simulink model "modello_completo_simulink2018b"  (R2018b)
settings: Solver=VariableStepAuto  StartTime=0.0  StopTime=10  RelTol=1e-3
undefined symbols (not defined in the file): a1, a2, AHRS_bias, AHRS_sample_time, AHRS_var, alpha1, alpha2, c, current, D, dead_zone_limit, DVL_sample_t, DVL_var1, DVL_var2, DVL_var3, gps_sample_t, IMU_sample_time, initial, M, M_inv, n_max, omega, ps_sample_t, ps_sample_t2, ps_var, ps_var2, pylonCenter, pylonRadius, rho, s_data, TAM
libraries: simulink x3
(part 1 of 2)
settings Model: Creator=andrea  LastModifiedBy=stefano
settings DataIOCC: ReturnWorkspaceOutputs=on

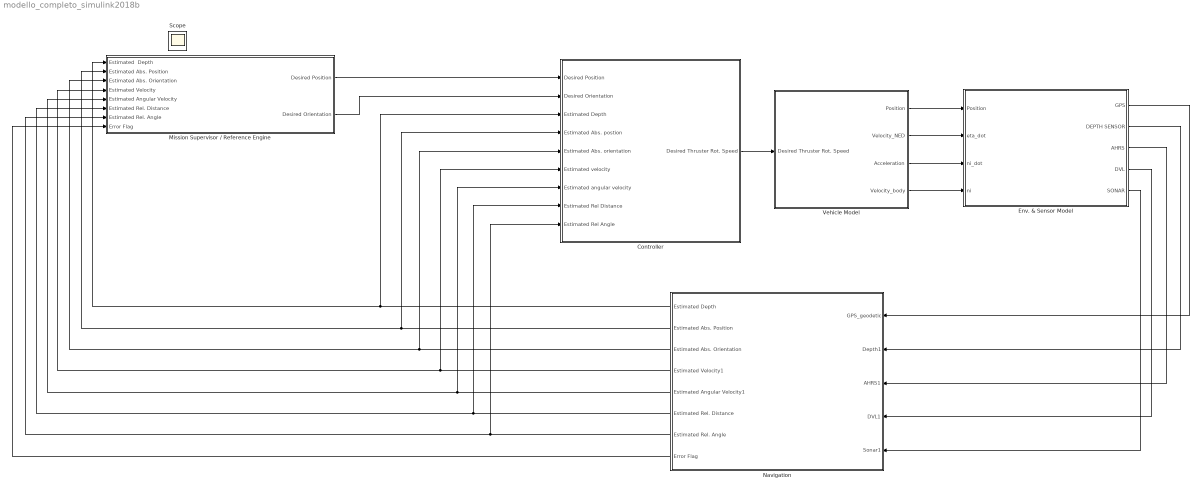
== system modello_completo_simulink2018b ==
  Controller : Subsystem
  Env. & Sensor Model : Subsystem
  Mission Supervisor / Reference Engine : Subsystem
  Navigation : Subsystem
  Vehicle Model : Subsystem
      mask Display: image('maronn17.jpg')
  Scope : Scope
  wires:
  Mission Supervisor / Reference Engine/1(Desired Position) -> Controller/1(Desired Position)
  Mission Supervisor / Reference Engine/2(Desired Orientation) -> Controller/2(Desired Orientation)
  Controller/1(Desired Thruster Rot. Speed) -> Vehicle Model/1(Desired Thruster Rot. Speed)
  Vehicle Model/1(Position) -> Env. & Sensor Model/1(Position)
  Env. & Sensor Model/1(GPS) -> Navigation/1(GPS_geodetic)
  Env. & Sensor Model/2(DEPTH SENSOR) -> Navigation/2(Depth1)
  Env. & Sensor Model/3(AHRS) -> Navigation/3(AHRS1)
  Env. & Sensor Model/4("DVL ") -> Navigation/4(DVL1)
  Env. & Sensor Model/5(SONAR) -> Navigation/5(Sonar1)
  Navigation/1(Estimated Depth) -> Mission Supervisor / Reference Engine/1(Estimated  Depth), Controller/3(Estimated Depth)
  Navigation/2(Estimated Abs. Position) -> Mission Supervisor / Reference Engine/2(Estimated Abs. Position), Controller/4(Estimated Abs. postion)
  Navigation/3(Estimated Abs. Orientation) -> Controller/5(Estimated Abs. orientation), Mission Supervisor / Reference Engine/3(Estimated Abs. Orientation)
  Navigation/4(Estimated Velocity1) -> Controller/6(Estimated velocity), Mission Supervisor / Reference Engine/4(Estimated Velocity)
  Vehicle Model/4(Velocity_body) -> Env. & Sensor Model/4(ni)
  Navigation/5(Estimated Angular Velocity1) -> Mission Supervisor / Reference Engine/5(Estimated Angular Velocity), Controller/7(Estimated angular velocity)
  Navigation/6(Estimated Rel. Distance) -> Mission Supervisor / Reference Engine/6(Estimated Rel. Distance), Controller/8(Estimated Rel Distance)
  Navigation/7(Estimated Rel. Angle) -> Mission Supervisor / Reference Engine/7(Estimated Rel. Angle), Controller/9(Estimated Rel Angle)
  Navigation/8(Error Flag) -> Mission Supervisor / Reference Engine/8(Error Flag)
  Vehicle Model/2(Velocity_NED) -> Env. & Sensor Model/2(eta_dot)
  Vehicle Model/3(Acceleration) -> Env. & Sensor Model/3(ni_dot)

== system modello_completo_simulink2018b/Controller ==
  note: Velocità dei thuster (rad/s)
  Desired Position : Inport
  Desired Orientation : Inport  Port=2
  Estimated Depth : Inport  Port=3
  Estimated Abs. postion : Inport  Port=4
  Estimated Abs. orientation : Inport  Port=5
  Estimated velocity : Inport  Port=6
  Estimated angular velocity : Inport  Port=7
  Estimated Rel Distance : Inport  Port=8
  Estimated Rel Angle : Inport  Port=9
  Desired Thruster Rot. Speed : Outport

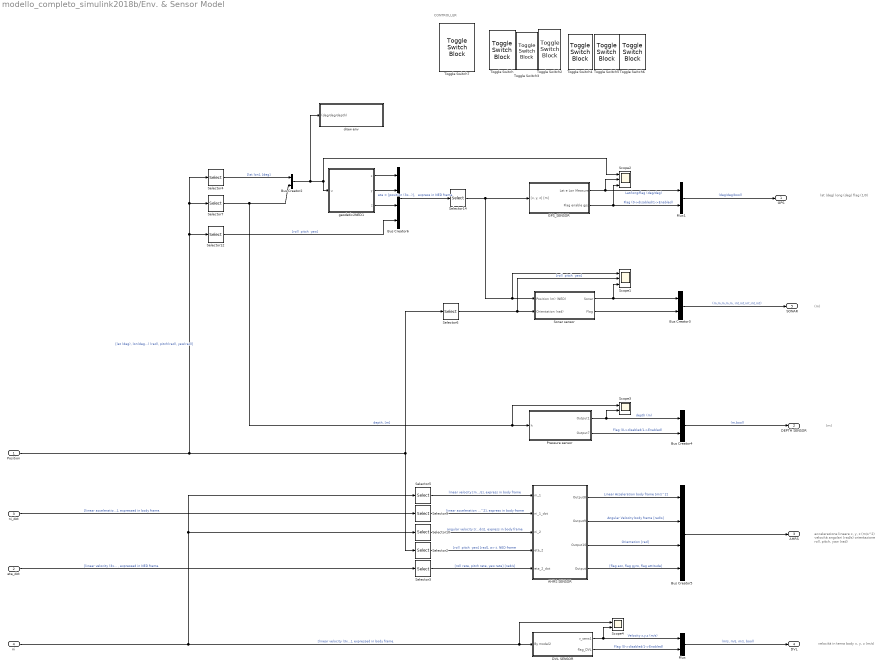
== system modello_completo_simulink2018b/Env. & Sensor Model ==
  note: (m)
  note: velocità in terna body x, y, z (m/s)
  note: accelerazione lineare x, y, z (m/s^2)
      | velocità angolari (rad/s)
      | orientazione roll, pitch, yaw (rad)
  note: (m)
  note: lat (deg)
      | long (deg)
      | flag (1/0)
  note: CONTROLLER
  Position : Inport
  eta_dot : Inport  Port=2
  ni_dot : Inport  Port=3
  ni : Inport  Port=4
  AHRS SENSOR : Subsystem
  Bus Creator2 : BusCreator  Inputs=2
  Bus Creator3 : BusCreator  Inputs=2
  Bus Creator4 : BusCreator  Inputs=2
  Bus Creator5 : BusCreator  Inputs=4
  Bus Creator6 : BusCreator  Inputs=4
  DVL SENSOR : Subsystem
  GPS_SENSOR : Subsystem
  Mux : Mux  Inputs=2
  Mux1 : Mux  Inputs=2
  Pressure sensor : Subsystem
  Scope1 : Scope  NumInputPorts=3
  Scope2 : Scope  NumInputPorts=3
  Scope3 : Scope  NumInputPorts=2
  Scope4 : Scope  NumInputPorts=2
  Selector{2..3,6,10,12} (5 alike) : Selector  InputPortWidth=6  IndexOptions=Index vector (dialog)  Indices=[4 5 6]  OutputSizes=1
  Selector14 : Selector  InputPortWidth=6  IndexOptions=Index vector (dialog)  Indices=[1 2 3]  OutputSizes=1
  Selector4 : Selector  InputPortWidth=6  IndexOptions=Index vector (dialog)  Indices=[1 2]  OutputSizes=1
  Selector5 : Selector  InputPortWidth=6  IndexOptions=Index vector (dialog)  Indices=[1 2 3]  OutputSizes=1
  Selector7 : Selector  InputPortWidth=6  IndexOptions=Index vector (dialog)  Indices=[3]  OutputSizes=1
  Selector9 : Selector  InputPortWidth=6  IndexOptions=Index vector (dialog)  Indices=[1 2 3]  OutputSizes=1
  Sonar sensor : Subsystem
  Toggle Switch : ToggleSwitchBlock  WebBlockId=1524
      settings: Values={{'Off', 'On'}, [0 1]}
  Toggle Switch2 : ToggleSwitchBlock  WebBlockId=1525
      settings: Values={{'Off', 'On'}, [0 1]}
  Toggle Switch3 : ToggleSwitchBlock  WebBlockId=1526
      settings: Values={{'Off', 'On'}, [0 1]}
  Toggle Switch4 : ToggleSwitchBlock  WebBlockId=1527
      settings: Values={{'Off', 'On'}, [0 1]}
  Toggle Switch5 : ToggleSwitchBlock  WebBlockId=1528
      settings: Values={{'Off', 'On'}, [0 1]}
  Toggle Switch6 : ToggleSwitchBlock  WebBlockId=1529
      settings: Values={{'Off', 'On'}, [0 1]}
  Toggle Switch7 : ToggleSwitchBlock  WebBlockId=1530
      settings: Values={{'Off', 'On'}, [0 1]}
  draw env : Subsystem
  geodetic2NED1 : MATLAB Function  TreatAsAtomicUnit=on
  GPS : Outport
  DEPTH SENSOR : Outport  Port=2
  AHRS : Outport  Port=3
  "DVL " : Outport  Port=4
  SONAR : Outport  Port=5
  wires:
  Pressure sensor/1(Output1) -> Bus Creator4/1, Scope3/2  "depth (m)"
  AHRS SENSOR/1(Output8) -> Bus Creator5/1  "Linear Acceleration body frame [m/s^2]"
  Mux1/1 -> GPS/1  "(deg/deg/bool)"
  AHRS SENSOR/3(Output10) -> Bus Creator5/3  "Orientation [rad]"
  Bus Creator6/1 -> Selector14/1  "eta = [position (3x1),  \t  orientation (3x1)], \t  express in NED frame."
  Selector14/1 -> GPS_SENSOR/1("[x, y, z] [m]"), Sonar sensor/1(Position (m) (NED)), Scope1/1
  GPS_SENSOR/1(Lat e Lon Measure) -> Scope2/2, Mux1/1  "Lat/long/flag (deg/deg)"
  Selector7/1 -> Pressure sensor/1(h), Scope3/1, Bus Creator2/2  "depth, [m]"
  geodetic2NED1/3(z) -> Bus Creator6/3
  Selector2/1 -> AHRS SENSOR/4(eta_2)  "[roll  pitch  yaw] [rad], w.r.t. NED frame"
  Bus Creator5/1 -> AHRS/1
  AHRS SENSOR/2(Output9) -> Bus Creator5/2  "Angular Velocity body frame [rad/s]"
  ni/1 -> DVL SENSOR/1(By model2), Scope4/1, Selector10/1, Selector5/1  "[linear velocity (3x1),angular velocity (3x1)], expressed in body frame."
  Selector6/1 -> Sonar sensor/2(Orientation (rad)), Scope1/2  "[roll  pitch  yaw]"
  AHRS SENSOR/4(Output) -> Bus Creator5/4  "[flag acc, flag gyro, flag attitude]"
  GPS_SENSOR/2(Flag enable gps) -> Scope2/3, Mux1/2  "Flag (0->disabled/1->Enabled)"
  Selector10/1 -> AHRS SENSOR/3(ni_2)  "angular velocity [rad/s], express in body frame"
  eta_dot/1 -> Selector3/1  "[linear velocity (3x1), roll rate, pitch rate, yaw rate] , expressed in NED frame."
  Selector9/1 -> AHRS SENSOR/2(ni_1_dot)  "linear acceleration [m/s^2], express in body frame"
  Pressure sensor/2(Output7) -> Bus Creator4/2  "Flag (0->disabled/1->Enabled)"
  Selector4/1 -> Bus Creator2/1  "[lat lon], [deg]"
  DVL SENSOR/2(flag_DVL) -> Mux/2  "Flag (0->disabled/1->Enabled)"
  Mux/1 -> "DVL "/1  "(m/s, m/s, m/s, bool)"
  geodetic2NED1/1(x) -> Bus Creator6/1
  geodetic2NED1/2(y) -> Bus Creator6/2
  Selector3/1 -> AHRS SENSOR/5(eta_2_dot)  "[roll rate, pitch rate, yaw rate] [rad/s]"
  Sonar sensor/1(Sonar) -> Scope1/3, Bus Creator3/1
  Position/1 -> Selector2/1, Selector6/1, Selector4/1, Selector7/1, Selector12/1  "[lat (deg), lon(deg), depth(m), roll (rad), pitch(rad), yaw(rad)]"
  Bus Creator4/1 -> DEPTH SENSOR/1  "(m,bool)"
  Selector5/1 -> AHRS SENSOR/1(ni_1)  "linear velocity [m/s], express in body frame"
  ni_dot/1 -> Selector9/1  "[linear acceleration (3x1), angular acceleration (3x1)], expressed in body frame."
  Bus Creator2/1 -> draw env/1((deg/deg/depth)), Scope2/1, geodetic2NED1/1(u)
  DVL SENSOR/1(v_sens1) -> Scope4/2, Mux/1  "Velocity x,y,z (m/s)"
  Bus Creator3/1 -> SONAR/1  "(m,m,m,m,m, int,int,int,int,int)"
  Sonar sensor/2(Flag) -> Bus Creator3/2
  Selector12/1 -> Bus Creator6/4  "[roll  pitch  yaw]"

== system modello_completo_simulink2018b/Mission Supervisor // Reference Engine ==
  note: Roll (rad): 0 == aligned with water surface
      | Pitch (rad): 0 == aligned with water surface
      | Yaw (rad): 0 == north
  note: Latitude (rad)
      | Longitude (rad)
      | Depth (m): 0 == water surface
  Estimated  Depth : Inport
  Estimated Abs. Position : Inport  Port=2
  Estimated Abs. Orientation : Inport  Port=3
  Estimated Velocity : Inport  Port=4
  Estimated Angular Velocity : Inport  Port=5
  Estimated Rel. Distance : Inport  Port=6
  Estimated Rel. Angle : Inport  Port=7
  Error Flag : Inport  Port=8
  Desired Position : Outport
  Desired Orientation : Outport  Port=2

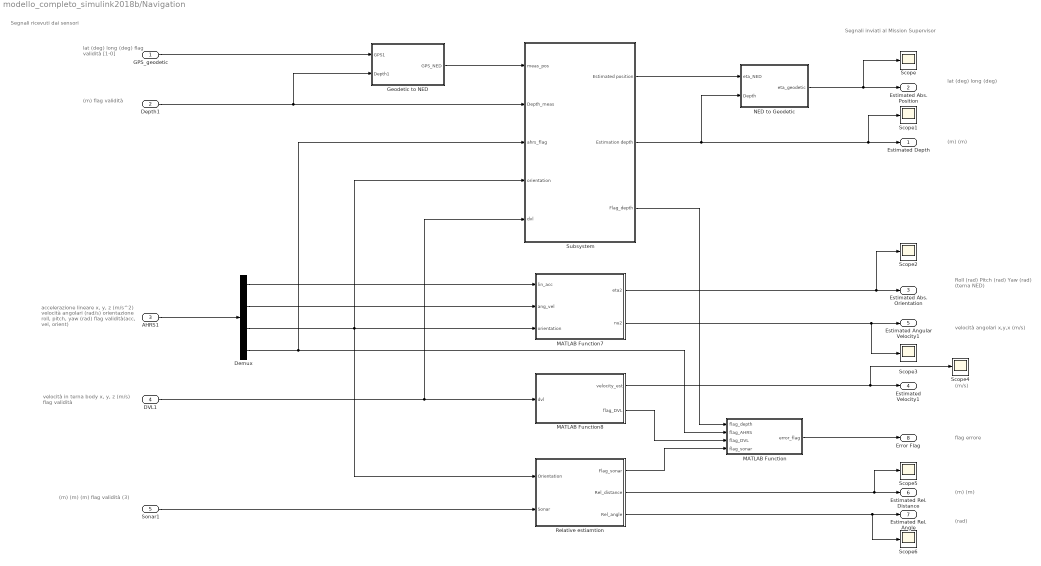
== system modello_completo_simulink2018b/Navigation ==
  note: Segnali inviati al Mission Supervisor
  note: velocità in terna body x, y, z (m/s)
      | flag validità
  note: (m)
      | flag validità
  note: (m)
      | (m)
      | (m)
      | flag validità (3)
  note: velocità angolari x,y,x (m/s)
  note: (m)
      | (m)
  note: (m)
      | (m)
  note: flag errore
  note: lat     (deg)
      |  long  (deg)
  note: lat     (deg)
      |  long  (deg)
      | flag validità [1-0]
  note: (m/s)
  note: Roll (rad)
      | Pitch (rad)
      | Yaw (rad)
      | (terna NED)
  note: (rad)
  note: accelerazione lineare x, y, z (m/s^2)
      | velocità angolari (rad/s)
      | orientazione roll, pitch, yaw (rad)
      | flag validità(acc, vel, orient)
  note: Segnali ricevuti dai sensori
  GPS_geodetic : Inport  PortDimensions=3
  Depth1 : Inport  Port=2  PortDimensions=2
  AHRS1 : Inport  Port=3  PortDimensions=12
  DVL1 : Inport  Port=4  PortDimensions=4
  Sonar1 : Inport  Port=5  PortDimensions=6
  Demux : Demux
  Geodetic to NED : Subsystem
  MATLAB Function : MATLAB Function  TreatAsAtomicUnit=on
  MATLAB Function7 : MATLAB Function  TreatAsAtomicUnit=on
  MATLAB Function8 : MATLAB Function  TreatAsAtomicUnit=on
  NED to Geodetic : Subsystem
  Relative estiamtion : Subsystem
  Scope{,1..6} (7 alike) : Scope
  Subsystem : Subsystem
  Estimated Depth : Outport
  Estimated Abs. Position : Outport  Port=2
  Estimated Abs. Orientation : Outport  Port=3
  Estimated Velocity1 : Outport  Port=4
  Estimated Angular Velocity1 : Outport  Port=5
  Estimated Rel. Distance : Outport  Port=6
  Estimated Rel. Angle : Outport  Port=7
  Error Flag : Outport  Port=8
  wires:
  Subsystem/2(Estimation depth) -> NED to Geodetic/2(Depth), Scope1/1, Estimated Depth/1
  Relative estiamtion/2(Rel_distance) -> Scope5/1, Estimated Rel. Distance/1
  MATLAB Function7/1(eta2) -> Scope2/1, Estimated Abs. Orientation/1
  Demux/4 -> Subsystem/3(ahrs_flag), MATLAB Function/2(flag_AHRS)
  Subsystem/3(Flag_depth) -> MATLAB Function/1(flag_depth)
  MATLAB Function8/2(flag_DVL) -> MATLAB Function/3(flag_DVL)
  NED to Geodetic/1(eta_geodetic) -> Scope/1, Estimated Abs. Position/1
  Geodetic to NED/1(GPS_NED) -> Subsystem/1(meas_pos)
  MATLAB Function/1(error_flag) -> Error Flag/1
  Demux/2 -> MATLAB Function7/2(ang_vel)
  DVL1/1 -> Subsystem/5(dvl), MATLAB Function8/1(dvl)
  Depth1/1 -> Subsystem/2(Depth_meas), Geodetic to NED/2(Depth1)
  GPS_geodetic/1 -> Geodetic to NED/1(GPS1)
  Sonar1/1 -> Relative estiamtion/2(Sonar)
  Subsystem/1(Estimated position) -> NED to Geodetic/1(eta_NED)
  Relative estiamtion/1(Flag_sonar) -> MATLAB Function/4(flag_sonar)
  Demux/3 -> MATLAB Function7/3(orientation), Relative estiamtion/1(Orientation), Subsystem/4(orientation)
  MATLAB Function7/2(nu2) -> Estimated Angular Velocity1/1, Scope3/1
  AHRS1/1 -> Demux/1
  Relative estiamtion/3(Rel_angle) -> Scope6/1, Estimated Rel. Angle/1
  MATLAB Function8/1(velocity_est) -> Scope4/1, Estimated Velocity1/1
  Demux/1 -> MATLAB Function7/1(lin_acc)

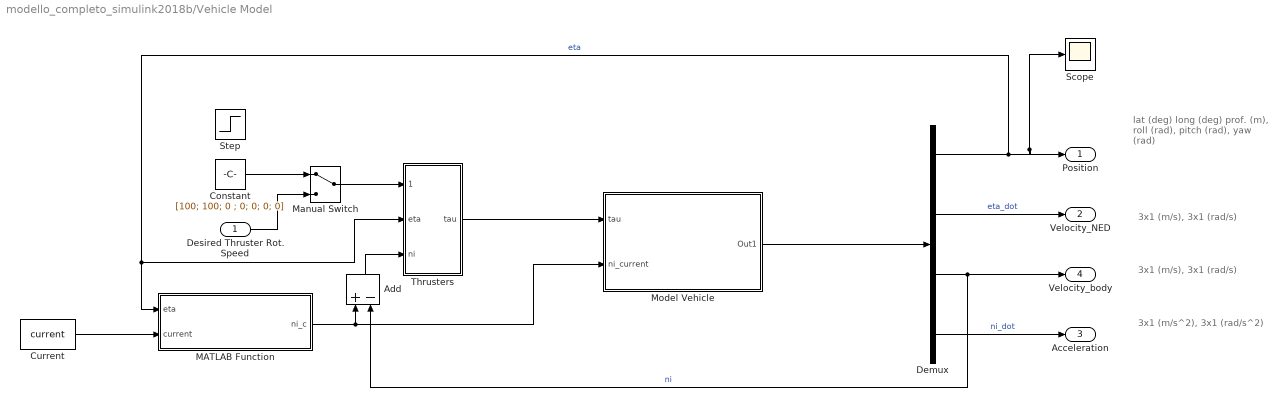
== system modello_completo_simulink2018b/Vehicle Model ==
  note: 3x1 (m/s^2),
      | 3x1 (rad/s^2)
  note: 3x1 (m/s),
      | 3x1 (rad/s)
  note: lat (deg)
      | long (deg)
      | prof. (m),
      | roll (rad),
      | pitch (rad),
      | yaw (rad)
  note: 3x1 (m/s),
      | 3x1 (rad/s)
  Desired Thruster Rot. Speed : Inport
  Add : Sum  Inputs=+-
  Constant : Constant  Value=[100; 100; 0 ; 0; 0; 0; 0]
  Current : Constant  Value=current
  Demux : Demux
  MATLAB Function : MATLAB Function  TreatAsAtomicUnit=on
  Manual Switch : ManualSwitch
  Model Vehicle : Subsystem
      mask Display: image('anna117.jpg')
  Scope : Scope
  Step : Step  Time=100  Before=[0;0;0;0;0;0;0]  After=[0;0;0;0;100;100;200]  SampleTime=0
  Thrusters : Subsystem
      mask Display: image('THRUSTER17.jpg')
  Position : Outport
  Velocity_NED : Outport  Port=2
  Acceleration : Outport  Port=3
  Velocity_body : Outport  Port=4
  wires:
  Demux/3 -> Velocity_body/1, Add/2  "ni"
  Model Vehicle/1(Out1) -> Demux/1
  Demux/1 -> Thrusters/2(eta), MATLAB Function/1(eta), Position/1, Scope/1  "eta"
  Desired Thruster Rot. Speed/1 -> Manual Switch/2
  Manual Switch/1 -> Thrusters/1(des rot)
  Current/1 -> MATLAB Function/2(current)
  Demux/2 -> Velocity_NED/1  "eta_dot"
  Demux/4 -> Acceleration/1  "ni_dot"
  MATLAB Function/1(ni_c) -> Model Vehicle/2(ni_current), Add/1
  Add/1 -> Thrusters/3(ni)
  Thrusters/1(tau) -> Model Vehicle/1(tau)
  Constant/1 -> Manual Switch/1

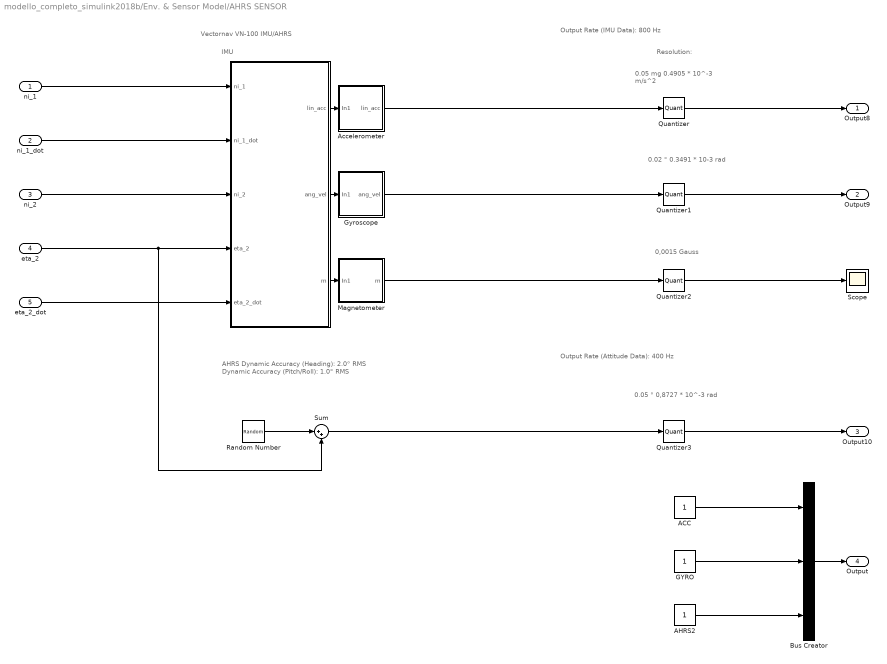
== system modello_completo_simulink2018b/Env. & Sensor Model/AHRS SENSOR ==
  note: AHRS
      |
      | Dynamic Accuracy (Heading):   2.0° RMS
      | Dynamic Accuracy (Pitch/Roll): 1.0° RMS
  note: Output Rate (IMU Data): 800 Hz
  note: Resolution:
  note: 0.02		      	 °
      | 0.3491 * 10-3 rad
  note: 0.05				°
      | 0,8727 * 10^-3	rad
  note: 0,0015 Gauss
  note: Vectornav VN-100 IMU/AHRS
  note: IMU
  note: 0.05			    mg
      | 0.4905 * 10^-3  m/s^2
  note: Output Rate (Attitude Data): 400 Hz
  ni_1 : Inport  SampleTime=IMU_sample_time
  ni_1_dot : Inport  Port=2  SampleTime=IMU_sample_time
  ni_2 : Inport  Port=3  SampleTime=IMU_sample_time
  eta_2 : Inport  Port=4  SampleTime=AHRS_sample_time
  eta_2_dot : Inport  Port=5  SampleTime=IMU_sample_time
  "   " : MATLAB Function  TreatAsAtomicUnit=on
  ACC : Constant
  AHRS2 : Constant
  Accelerometer : Subsystem
  Bus Creator : BusCreator  Inputs=3
  GYRO : Constant
  Gyroscope : Subsystem
  Magnetometer : Subsystem
  Quantizer : Quantizer  QuantizationInterval=Resolution_acc
  Quantizer1 : Quantizer  QuantizationInterval=Resolution_gyro
  Quantizer2 : Quantizer  QuantizationInterval=Resolution_magn
  Quantizer3 : Quantizer  QuantizationInterval=Resolution_AHRS
  Random Number : RandomNumber  Mean=AHRS_bias  Variance=AHRS_var  Seed=[232 342 202]  SampleTime=AHRS_sample_time
  Scope : Scope
  Sum : Sum  Inputs=|++
  Output8 : Outport  SampleTime=IMU_sample_time
  Output9 : Outport  Port=2  SampleTime=IMU_sample_time
  Output10 : Outport  Port=3  SampleTime=AHRS_sample_time
  Output : Outport  Port=4
  wires:
  "   "/2(ang_vel) -> Gyroscope/1(In1)
  Gyroscope/1(ang_vel) -> Quantizer1/1
  ni_1/1 -> "   "/1(ni_1)
  eta_2/1 -> Sum/2, "   "/4(eta_2)
  ni_2/1 -> "   "/3(ni_2)
  Quantizer2/1 -> Scope/1
  Quantizer1/1 -> Output9/1
  Accelerometer/1(lin_acc) -> Quantizer/1
  ni_1_dot/1 -> "   "/2(ni_1_dot)
  Sum/1 -> Quantizer3/1
  "   "/1(lin_acc) -> Accelerometer/1(In1)
  Quantizer/1 -> Output8/1
  eta_2_dot/1 -> "   "/5(eta_2_dot)
  Random Number/1 -> Sum/1
  "   "/3(m) -> Magnetometer/1(In1)
  Magnetometer/1(m) -> Quantizer2/1
  Quantizer3/1 -> Output10/1
  ACC/1 -> Bus Creator/1
  GYRO/1 -> Bus Creator/2
  AHRS2/1 -> Bus Creator/3
  Bus Creator/1 -> Output/1

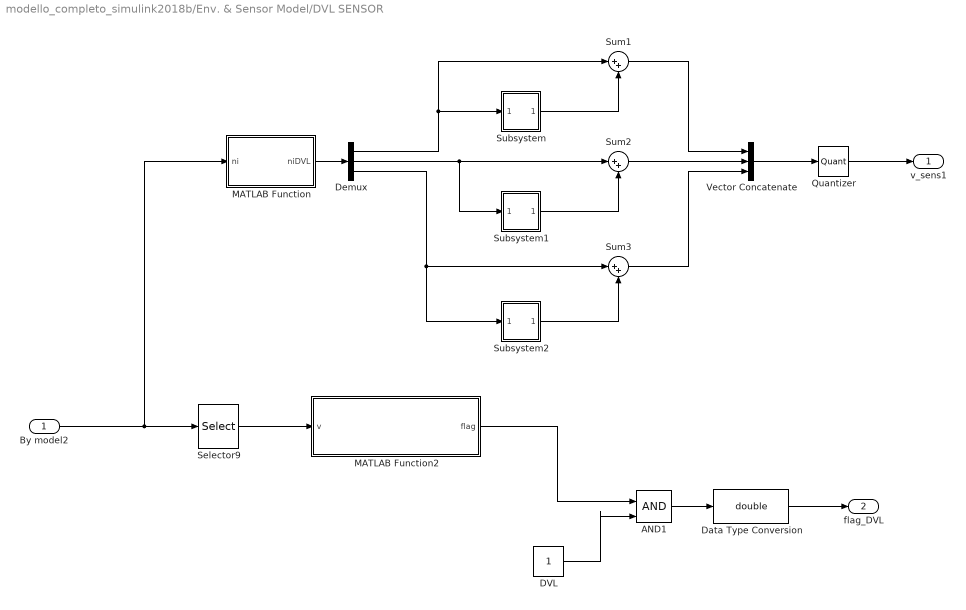
== system modello_completo_simulink2018b/Env. & Sensor Model/DVL SENSOR ==
  By model2 : Inport  SampleTime=DVL_sample_t
  AND1 : Logic  IconShape=distinctive  AllPortsSameDT=off  OutDataTypeStr=boolean
  DVL : Constant
  Data Type Conversion : DataTypeConversion  OutDataTypeStr=double
  Demux : Demux  Outputs=3
  MATLAB Function : MATLAB Function  TreatAsAtomicUnit=on
  MATLAB Function2 : MATLAB Function  TreatAsAtomicUnit=on
  Quantizer : Quantizer  QuantizationInterval=DVL_resol
  Selector9 : Selector  InputPortWidth=6  IndexOptions=Index vector (dialog)  Indices=[1 2 3]  OutputSizes=1
  Subsystem : Subsystem
  Subsystem1 : Subsystem
  Subsystem2 : Subsystem
  Sum1 : Sum  Inputs=|++
  Sum2 : Sum  Inputs=|++
  Sum3 : Sum  Inputs=|++
  Vector Concatenate : Concatenate  NumInputs=3
  v_sens1 : Outport  SampleTime=DVL_sample_t
  flag_DVL : Outport  Port=2  SampleTime=DVL_sample_t
  wires:
  MATLAB Function2/1(flag) -> AND1/1
  DVL/1 -> AND1/2
  AND1/1 -> Data Type Conversion/1
  Demux/1 -> Sum1/1, Subsystem/1(In1)
  Subsystem/1(Out1) -> Sum1/2
  Demux/2 -> Sum2/1, Subsystem1/1(In1)
  Subsystem1/1(Out1) -> Sum2/2
  Demux/3 -> Sum3/1, Subsystem2/1(In1)
  Subsystem2/1(Out1) -> Sum3/2
  Sum2/1 -> Vector Concatenate/2
  Sum1/1 -> Vector Concatenate/1
  Sum3/1 -> Vector Concatenate/3
  Vector Concatenate/1 -> Quantizer/1
  By model2/1 -> MATLAB Function/1(ni), Selector9/1
  Quantizer/1 -> v_sens1/1
  Data Type Conversion/1 -> flag_DVL/1
  Selector9/1 -> MATLAB Function2/1(v)
  MATLAB Function/1(niDVL) -> Demux/1

== system modello_completo_simulink2018b/Env. & Sensor Model/GPS_SENSOR ==
  note: Copernicus II DIP
  note: Control state sensors. 1:enabled, 0:disabled
  "[x, y, z] [m]" : Inport  SampleTime=gps_sample_t
  Add noiose : Subsystem
  Control state : Subsystem
  Demux : Demux  Outputs=3
  NED2Geodetic : MATLAB Function  TreatAsAtomicUnit=on
  Threshold : MATLAB Function  TreatAsAtomicUnit=on
  Zero-Order Hold : ZeroOrderHold  SampleTime=gps_sample_t
  Lat e Lon Measure : Outport
  Flag enable gps : Outport  Port=2
  wires:
  Threshold/2(x_out) -> Add noiose/1(In1)  "x"
  Threshold/3(y_out) -> Add noiose/2(In2)  "y"
  Threshold/1(depth) -> NED2Geodetic/1(depth)
  Add noiose/1(Out1) -> NED2Geodetic/2(u)  "out"
  Threshold/4(flag_enable_gps) -> Control state/1(In1)
  Control state/1(Flag enable gps) -> NED2Geodetic/3(enableGps), Flag enable gps/1
  NED2Geodetic/1(data_GDT) -> Zero-Order Hold/1
  "[x, y, z] [m]"/1 -> Demux/1
  Demux/1 -> Threshold/1(x_in)
  Demux/2 -> Threshold/2(y_in)
  Demux/3 -> Threshold/3(h_in)
  Zero-Order Hold/1 -> Lat e Lon Measure/1  "(deg/deg/bool)"

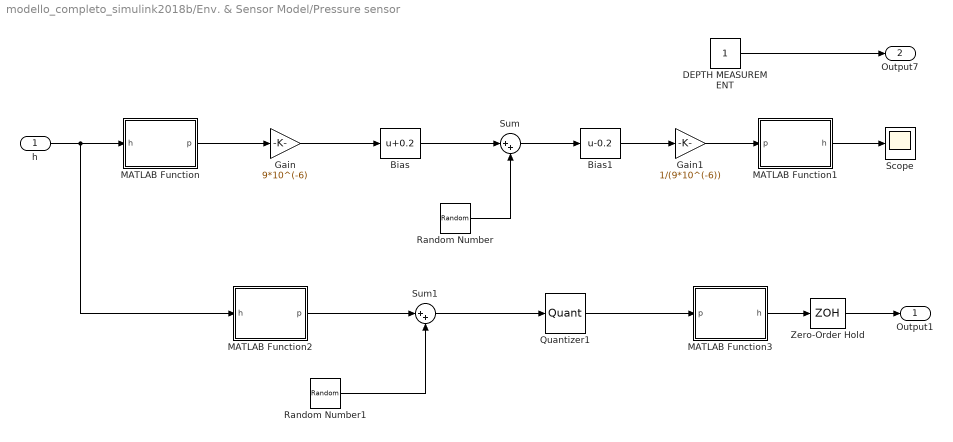
== system modello_completo_simulink2018b/Env. & Sensor Model/Pressure sensor ==
  h : Inport  SampleTime=ps_sample_t
  Bias : Bias  Bias=0.2
  Bias1 : Bias  Bias=-0.2
  DEPTH MEASUREMENT : Constant  SampleTime=ps_sample_t
  Gain : Gain  Gain=9*10^(-6)
  Gain1 : Gain  Gain=1/(9*10^(-6))
  MATLAB Function : MATLAB Function  TreatAsAtomicUnit=on
  MATLAB Function1 : MATLAB Function  TreatAsAtomicUnit=on
  MATLAB Function2 : MATLAB Function  TreatAsAtomicUnit=on
  MATLAB Function3 : MATLAB Function  TreatAsAtomicUnit=on
  Quantizer1 : Quantizer  QuantizationInterval=ps_resol  LinearizeAsGain=off
  Random Number : RandomNumber  Variance=ps_var2  SampleTime=ps_sample_t2
  Random Number1 : RandomNumber  Variance=ps_var  SampleTime=ps_sample_t
  Scope : Scope
  Sum : Sum  Inputs=|++
  Sum1 : Sum  Inputs=|++
  Zero-Order Hold : ZeroOrderHold  SampleTime=ps_sample_t
  Output1 : Outport  SampleTime=ps_sample_t
  Output7 : Outport  Port=2  SampleTime=ps_sample_t
  wires:
  Bias/1 -> Sum/1
  MATLAB Function/1(p) -> Gain/1
  Gain/1 -> Bias/1
  Gain1/1 -> MATLAB Function1/1(p)
  MATLAB Function1/1(h) -> Scope/1
  Sum/1 -> Bias1/1
  Bias1/1 -> Gain1/1
  DEPTH MEASUREMENT/1 -> Output7/1
  Random Number/1 -> Sum/2
  Random Number1/1 -> Sum1/2
  MATLAB Function2/1(p) -> Sum1/1
  MATLAB Function3/1(h) -> Zero-Order Hold/1
  Sum1/1 -> Quantizer1/1
  Quantizer1/1 -> MATLAB Function3/1(p)
  h/1 -> MATLAB Function2/1(h), MATLAB Function/1(h)
  Zero-Order Hold/1 -> Output1/1

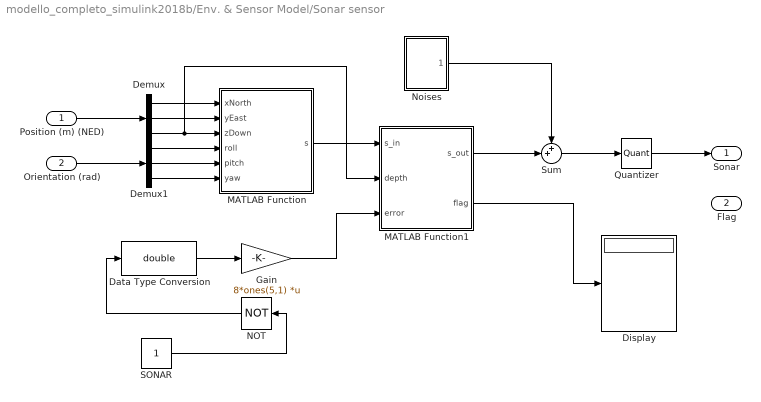
== system modello_completo_simulink2018b/Env. & Sensor Model/Sonar sensor ==
  Position (m) (NED) : Inport  SampleTime=s_data.smpl
  Orientation (rad) : Inport  Port=2  SampleTime=s_data.smpl
  Data Type Conversion : DataTypeConversion  OutDataTypeStr=double
  Demux : Demux  Outputs=3
  Demux1 : Demux  Outputs=3
  Display : Display
  Gain : Gain  Gain=8*ones(5,1)  Multiplication=Matrix(K*u)
  MATLAB Function : MATLAB Function  TreatAsAtomicUnit=on
  MATLAB Function1 : MATLAB Function  TreatAsAtomicUnit=on
  NOT : Logic  Operator=NOT  IconShape=distinctive  AllPortsSameDT=off  OutDataTypeStr=boolean
  Noises : Subsystem
  Quantizer : Quantizer  QuantizationInterval=s_data.res
  SONAR : Constant
  Sum : Sum  Inputs=++|
  Sonar : Outport
  Flag : Outport  Port=2
  wires:
  MATLAB Function/1(s) -> MATLAB Function1/1(s_in)
  MATLAB Function1/1(s_out) -> Sum/2
  Noises/1(Noises) -> Sum/1
  Position (m) (NED)/1 -> Demux/1
  Demux/1 -> MATLAB Function/1(xNorth)
  Demux/2 -> MATLAB Function/2(yEast)
  Demux/3 -> MATLAB Function1/2(depth), MATLAB Function/3(zDown)
  Demux1/3 -> MATLAB Function/6(yaw)
  Demux1/2 -> MATLAB Function/5(pitch)
  Demux1/1 -> MATLAB Function/4(roll)
  Orientation (rad)/1 -> Demux1/1
  Data Type Conversion/1 -> Gain/1
  Gain/1 -> MATLAB Function1/3(error)
  Quantizer/1 -> Sonar/1
  SONAR/1 -> NOT/1
  NOT/1 -> Data Type Conversion/1
  MATLAB Function1/2(flag) -> Display/1
  Sum/1 -> Quantizer/1

== system modello_completo_simulink2018b/Env. & Sensor Model/draw env ==
  (deg/deg/depth) : Inport
  DRAW ENV : Constant  Value=0
  MATLAB Function : MATLAB Function  TreatAsAtomicUnit=on
  wires:
  (deg/deg/depth)/1 -> MATLAB Function/2(u)
  DRAW ENV/1 -> MATLAB Function/1(enable_from_simulink)

== system modello_completo_simulink2018b/Navigation/Geodetic to NED ==
  GPS1 : Inport
  Depth1 : Inport  Port=2
  Demux : Demux  Outputs=2
  Demux1 : Demux  Outputs=[2 1]
  Gain1 : Gain  Gain=pi/180
  MATLAB Function2 : MATLAB Function  TreatAsAtomicUnit=on
  Terminator : Terminator
  GPS_NED : Outport
  wires:
  Demux1/2 -> MATLAB Function2/2(GPS_flag)
  MATLAB Function2/1(GPS_NED) -> GPS_NED/1
  GPS1/1 -> Demux1/1
  Demux1/1 -> Gain1/1
  Gain1/1 -> MATLAB Function2/1(GPS_geodetic)
  Depth1/1 -> Demux/1
  Demux/1 -> MATLAB Function2/3(depth)
  Demux/2 -> Terminator/1

== system modello_completo_simulink2018b/Navigation/NED to Geodetic ==
  eta_NED : Inport
  Depth : Inport  Port=2
  Gain : Gain  Gain=180/pi
  MATLAB Function1 : MATLAB Function  TreatAsAtomicUnit=on
  eta_geodetic : Outport  PortDimensions=2
  wires:
  Gain/1 -> eta_geodetic/1
  eta_NED/1 -> MATLAB Function1/1(eta_NED)
  MATLAB Function1/1(eta_geodetic) -> Gain/1
  Depth/1 -> MATLAB Function1/2(depth)

== system modello_completo_simulink2018b/Navigation/Relative estiamtion ==
  Orientation : Inport
  Sonar : Inport  Port=2
  Sonar trigger : Subsystem
  Subsystem : Subsystem
  Flag_sonar : Outport
  Rel_distance : Outport  Port=2
  Rel_angle : Outport  Port=3
  wires:
  Sonar/1 -> Sonar trigger/1(In1), Subsystem/1(Sonar)
  Sonar trigger/1(Out2) -> Subsystem/Trigger
  Orientation/1 -> Subsystem/2(Orientation)
  Subsystem/1(Rel_distance) -> Rel_distance/1
  Subsystem/2(Rel_angle) -> Rel_angle/1
  Subsystem/3(flag_sonar) -> Flag_sonar/1

== system modello_completo_simulink2018b/Navigation/Subsystem ==
  meas_pos : Inport
  Depth_meas : Inport  Port=2
  ahrs_flag : Inport  Port=3
  orientation : Inport  Port=4
  dvl : Inport  Port=5
  Demux1 : Demux  Outputs=[2 1]
  Demux2 : Demux  Outputs=[2 1]
  EKF : Subsystem  TreatAsAtomicUnit=on
  Terminator : Terminator
  Trigger & Init : Subsystem
  Estimated position : Outport
  Estimation depth : Outport  Port=2
  Flag_depth : Outport  Port=3
  wires:
  Trigger & Init/1(pulse) -> EKF/Trigger
  Trigger & Init/2(dT) -> EKF/1(dT)
  Demux2/1 -> EKF/6(meas_pos)
  orientation/1 -> EKF/9(orientation)
  meas_pos/1 -> Demux2/1, Trigger & Init/2("meas_pos ")
  Trigger & Init/6(P0_depth) -> EKF/5(P0_depth)
  Trigger & Init/3(init_pos) -> EKF/2(init_pos)
  Depth_meas/1 -> EKF/8(depth_meas), Trigger & Init/1(meas_depth)
  Demux2/2 -> EKF/7(GPS_flag)
  Trigger & Init/5(init_depth) -> EKF/4(init_depth)
  Trigger & Init/4(P0_pos) -> EKF/3(P0_pos)
  dvl/1 -> EKF/10(dvl)
  EKF/3(flag_depth) -> Flag_depth/1
  EKF/2(hat_depth) -> Estimation depth/1
  EKF/1(hat_pos) -> Estimated position/1
  ahrs_flag/1 -> Demux1/1
  Demux1/1 -> Terminator/1
  Demux1/2 -> EKF/11(orientation_flag)

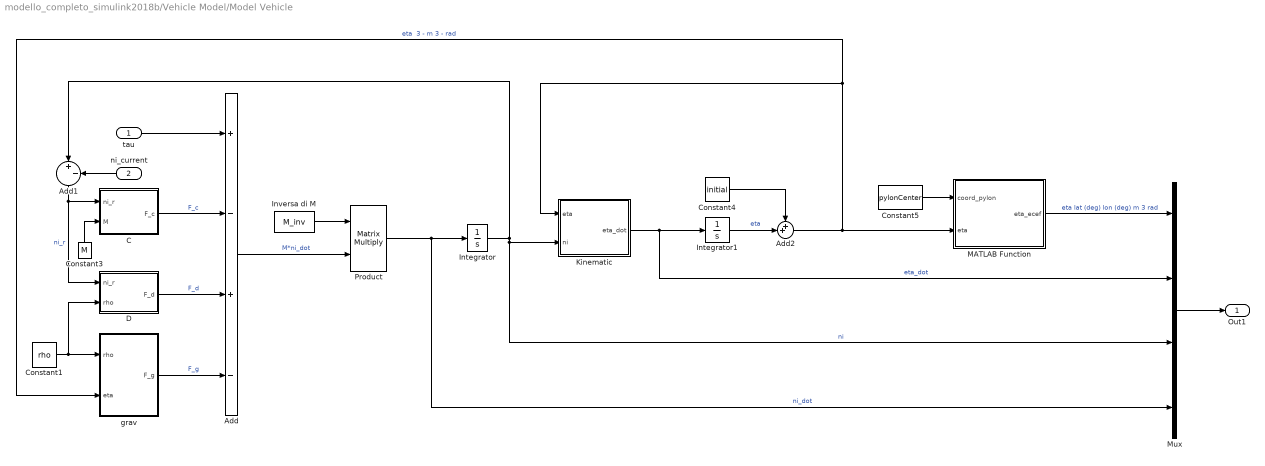
== system modello_completo_simulink2018b/Vehicle Model/Model Vehicle ==
  tau : Inport
  ni_current : Inport  Port=2
  Add : Sum  Inputs=+-+-
  Add1 : Sum  Inputs=|+-
  Add2 : Sum  Inputs=++|
  C : MATLAB Function  TreatAsAtomicUnit=on
  Constant1 : Constant  Value=rho
  Constant3 : Constant  Value=M
  Constant4 : Constant  Value=initial
  Constant5 : Constant  Value=pylonCenter
  D : MATLAB Function  TreatAsAtomicUnit=on
  Integrator : Integrator
  Integrator1 : Integrator
  Inversa di M : Constant  Value=M_inv
  Kinematic : Subsystem
      mask Display: image('herbert17.jpg')
  MATLAB Function : MATLAB Function  TreatAsAtomicUnit=on
  Mux : Mux
  Product : Product  Multiplication=Matrix(*)
  grav : MATLAB Function  TreatAsAtomicUnit=on
  Out1 : Outport  VectorParamsAs1DForOutWhenUnconnected=off
  wires:
  tau/1 -> Add/1
  Product/1 -> Mux/4, Integrator/1  "ni_dot"
  Integrator/1 -> Kinematic/2(ni), Mux/3, Add1/1  "ni"
  ni_current/1 -> Add1/2
  Add1/1 -> D/1(ni_r), C/1(ni_r)  "ni_r"
  Mux/1 -> Out1/1
  C/1(F_c) -> Add/2  "F_c"
  grav/1(F_g) -> Add/4  "F_g"
  Kinematic/1(eta_dot) -> Mux/2, Integrator1/1  "eta_dot"
  Inversa di M/1 -> Product/1
  Add/1 -> Product/2  "M*ni_dot"
  Constant1/1 -> grav/1(rho), D/2(rho)
  Constant3/1 -> C/2(M)
  D/1(F_d) -> Add/3  "F_d"
  Add2/1 -> MATLAB Function/2(eta), grav/2(eta), Kinematic/1(eta)  "eta  3 - m 3 - rad"
  MATLAB Function/1(eta_ecef) -> Mux/1  "eta lat (deg) lon (deg) m 3 rad"
  Constant5/1 -> MATLAB Function/1(coord_pylon)
  Constant4/1 -> Add2/1
  Integrator1/1 -> Add2/2  "eta"

== system modello_completo_simulink2018b/Vehicle Model/Thrusters ==
  des rot : Inport
  eta : Inport  Port=2
  ni : Inport  Port=3
  Product : Product  Multiplication=Matrix(*)
  T : Subsystem
      mask Display: image('download17.jpg')
  TAM : Constant  Value=TAM
  saturation_tau : MATLAB Function  TreatAsAtomicUnit=on
  tau : Outport  VectorParamsAs1DForOutWhenUnconnected=off
  wires:
  Product/1 -> saturation_tau/1(tau)
  des rot/1 -> T/1(des rot)
  TAM/1 -> Product/1
  T/1(T) -> Product/2
  saturation_tau/1(tau_sat) -> tau/1
  ni/1 -> T/2(ni)
  eta/1 -> saturation_tau/2(eta)

== system modello_completo_simulink2018b/Env. & Sensor Model/AHRS SENSOR/Accelerometer ==
  note: Noise Density: < 0.14 mg/√Hz
  In1 : Inport
  Band-Limited White Noise : simulink/Sources/Band-Limited White Noise  Cov=acc_noise  Ts=IMU_sample_time  seed=[23341]
  Bias : Bias  Bias=0.0
  Sum : Sum  Inputs=|++
  lin_acc : Outport
  wires:
  Band-Limited White Noise/1 -> Sum/2
  Sum/1 -> lin_acc/1
  Bias/1 -> Sum/1
  In1/1 -> Bias/1

== system modello_completo_simulink2018b/Env. & Sensor Model/AHRS SENSOR/Gyroscope ==
  note: Noise Density: 0.0035 °/s √Hz
  In1 : Inport
  Band-Limited White Noise : simulink/Sources/Band-Limited White Noise  Cov=gyro_noise  Ts=IMU_sample_time  seed=[341]
  Bias : Bias  Bias=0.0
  Sum : Sum  Inputs=|++
  ang_vel : Outport
  wires:
  Band-Limited White Noise/1 -> Sum/2
  Sum/1 -> ang_vel/1
  Bias/1 -> Sum/1
  In1/1 -> Bias/1

== system modello_completo_simulink2018b/Env. & Sensor Model/AHRS SENSOR/Magnetometer ==
  note: Noise Density: 140 μGauss/√Hz
  In1 : Inport
  Band-Limited White Noise : simulink/Sources/Band-Limited White Noise  Cov=magn_noise  Ts=IMU_sample_time  seed=[31]
  Bias : Bias  Bias=0.0
  Sum : Sum  Inputs=|++
  m : Outport
  wires:
  Band-Limited White Noise/1 -> Sum/2
  Sum/1 -> m/1
  Bias/1 -> Sum/1
  In1/1 -> Bias/1

== system modello_completo_simulink2018b/Env. & Sensor Model/DVL SENSOR/Subsystem ==
  In1 : Inport
  Random Number : RandomNumber  Variance=DVL_var3  Seed=1  SampleTime=DVL_sample_t
  Random Number1 : RandomNumber  Variance=DVL_var2  Seed=2  SampleTime=DVL_sample_t
  Random Number2 : RandomNumber  Variance=DVL_var1  Seed=3  SampleTime=DVL_sample_t
  Switch2 : Switch  Criteria=u2 > Threshold  Threshold=2
  Switch3 : Switch  Criteria=u2 > Threshold  Threshold=4
  Out1 : Outport
  wires:
  Switch3/1 -> Switch2/1
  Random Number1/1 -> Switch3/3
  Random Number2/1 -> Switch2/3
  In1/1 -> Switch3/2, Switch2/2
  Switch2/1 -> Out1/1
  Random Number/1 -> Switch3/1

== system modello_completo_simulink2018b/Env. & Sensor Model/DVL SENSOR/Subsystem1 ==
  In1 : Inport
  Random Number : RandomNumber  Variance=DVL_var3  Seed=4  SampleTime=DVL_sample_t
  Random Number1 : RandomNumber  Variance=DVL_var2  Seed=5  SampleTime=DVL_sample_t
  Random Number2 : RandomNumber  Variance=DVL_var1  Seed=2  SampleTime=DVL_sample_t
  Switch2 : Switch  Criteria=u2 > Threshold  Threshold=2
  Switch3 : Switch  Criteria=u2 > Threshold  Threshold=4
  Out1 : Outport
  wires:
  Switch3/1 -> Switch2/1
  Random Number1/1 -> Switch3/3
  Random Number2/1 -> Switch2/3
  In1/1 -> Switch3/2, Switch2/2
  Switch2/1 -> Out1/1
  Random Number/1 -> Switch3/1

== system modello_completo_simulink2018b/Env. & Sensor Model/DVL SENSOR/Subsystem2 ==
  In1 : Inport
  Random Number : RandomNumber  Variance=DVL_var3  Seed=7  SampleTime=DVL_sample_t
  Random Number1 : RandomNumber  Variance=DVL_var2  Seed=2  SampleTime=DVL_sample_t
  Random Number2 : RandomNumber  Variance=DVL_var1  Seed=1  SampleTime=DVL_sample_t
  Switch2 : Switch  Criteria=u2 > Threshold  Threshold=2
  Switch3 : Switch  Criteria=u2 > Threshold  Threshold=4
  Out1 : Outport
  wires:
  Switch3/1 -> Switch2/1
  Random Number1/1 -> Switch3/3
  Random Number2/1 -> Switch2/3
  In1/1 -> Switch3/2, Switch2/2
  Switch2/1 -> Out1/1
  Random Number/1 -> Switch3/1

== system modello_completo_simulink2018b/Env. & Sensor Model/GPS_SENSOR/Add noiose ==
  In1 : Inport
  In2 : Inport  Port=2
  Bus Creator : BusCreator  Inputs=2
  Random Number : RandomNumber  Variance=2  SampleTime=1
  Random Number1 : RandomNumber  Variance=2  Seed=332  SampleTime=1
  Sum2 : Sum  Inputs=|++
  Sum3 : Sum  Inputs=|++
  Out1 : Outport
  wires:
  In2/1 -> Sum3/1  "y in"
  Bus Creator/1 -> Out1/1  "out"
  In1/1 -> Sum2/1  "x in"
  Random Number/1 -> Sum2/2  "noise x"
  Random Number1/1 -> Sum3/2  "noise y"
  Sum2/1 -> Bus Creator/1  "x out"
  Sum3/1 -> Bus Creator/2  "y out"

== system modello_completo_simulink2018b/Env. & Sensor Model/GPS_SENSOR/Control state ==
  In1 : Inport
  AND : Logic  IconShape=distinctive  AllPortsSameDT=off  OutDataTypeStr=boolean
  Data Type Conversion : DataTypeConversion  OutDataTypeStr=double
  ENABLE GPS : Constant
  Zero-Order Hold : ZeroOrderHold  SampleTime=gps_sample_t
  Flag enable gps : Outport
  wires:
  ENABLE GPS/1 -> AND/2
  In1/1 -> AND/1
  AND/1 -> Data Type Conversion/1
  Data Type Conversion/1 -> Zero-Order Hold/1
  Zero-Order Hold/1 -> Flag enable gps/1

== system modello_completo_simulink2018b/Env. & Sensor Model/Sonar sensor/Noises ==
  Mux : Mux  Inputs=s_data.num
  Random Number : RandomNumber  Mean=s_data.bias  Variance=s_data.noise^2  Seed=1  SampleTime=s_data.smpl  VectorParams1D=off
  Random Number1 : RandomNumber  Mean=s_data.bias  Variance=s_data.noise^2  Seed=2  SampleTime=s_data.smpl  VectorParams1D=off
  Random Number2 : RandomNumber  Mean=s_data.bias  Variance=s_data.noise^2  Seed=3  SampleTime=s_data.smpl  VectorParams1D=off
  Random Number3 : RandomNumber  Mean=s_data.bias  Variance=s_data.noise^2  Seed=4  SampleTime=s_data.smpl  VectorParams1D=off
  Random Number4 : RandomNumber  Mean=s_data.bias  Variance=s_data.noise^2  Seed=5  SampleTime=s_data.smpl  VectorParams1D=off
  Noises : Outport
  wires:
  Mux/1 -> Noises/1
  Random Number/1 -> Mux/1
  Random Number1/1 -> Mux/2
  Random Number2/1 -> Mux/3
  Random Number3/1 -> Mux/4
  Random Number4/1 -> Mux/5

== system modello_completo_simulink2018b/Navigation/Relative estiamtion/Sonar trigger ==
  In1 : Inport
  Demux : Demux  Outputs=[3 3]
  MATLAB Function : MATLAB Function  TreatAsAtomicUnit=on  SystemSampleTime=1/200
  Scope2 : Scope
  Sum : Sum  Inputs=|+-
  Terminator : Terminator
  prev_sonar : Memory  InitialCondition=zeros(3,1)
  Out2 : Outport
  wires:
  Sum/1 -> MATLAB Function/2(sum)
  prev_sonar/1 -> Sum/2
  MATLAB Function/1(pulse) -> Out2/1, Scope2/1
  Demux/2 -> Terminator/1
  MATLAB Function/2(prev) -> prev_sonar/1
  In1/1 -> Demux/1
  Demux/1 -> MATLAB Function/1(sonar), Sum/1

== system modello_completo_simulink2018b/Navigation/Relative estiamtion/Subsystem ==
  Sonar : Inport
  Orientation : Inport  Port=2
  Trigger : TriggerPort  VariantControl=Variant  PortDimensions=1
  MATLAB Function9 : MATLAB Function  TreatAsAtomicUnit=on
  Rel_distance : Outport  PortDimensions=1
  Rel_angle : Outport  Port=2  PortDimensions=1
  flag_sonar : Outport  Port=3  PortDimensions=1
  wires:
  Sonar/1 -> MATLAB Function9/1(sonar)
  MATLAB Function9/3(flag_sonar) -> flag_sonar/1
  Orientation/1 -> MATLAB Function9/2(orientation)
  MATLAB Function9/2(alpha) -> Rel_angle/1
  MATLAB Function9/1(distance) -> Rel_distance/1

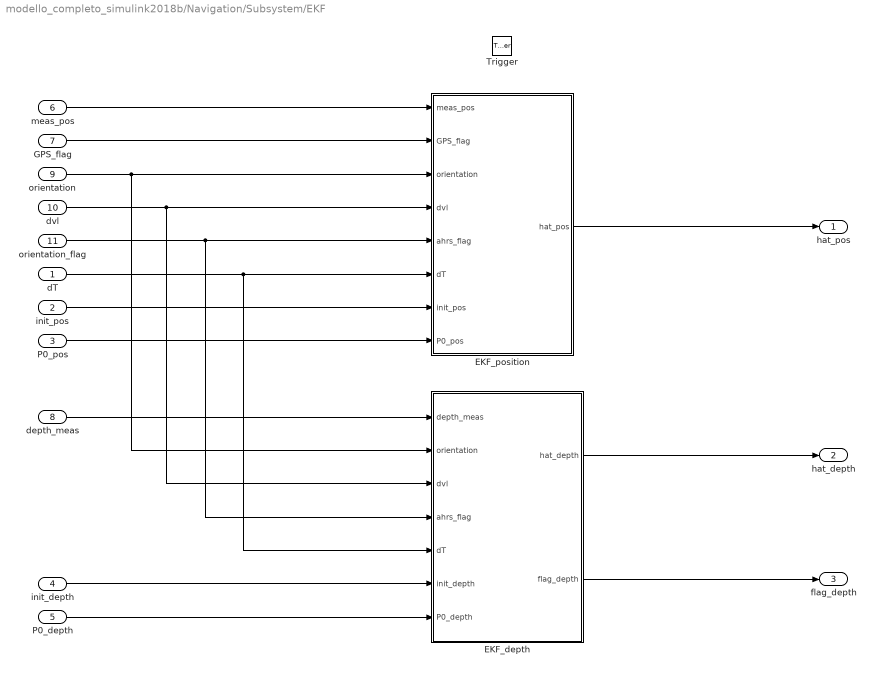
== system modello_completo_simulink2018b/Navigation/Subsystem/EKF ==
  dT : Inport
  init_pos : Inport  Port=2
  P0_pos : Inport  Port=3
  init_depth : Inport  Port=4
  P0_depth : Inport  Port=5
  meas_pos : Inport  Port=6
  GPS_flag : Inport  Port=7
  depth_meas : Inport  Port=8
  orientation : Inport  Port=9
  dvl : Inport  Port=10
  orientation_flag : Inport  Port=11
  Trigger : TriggerPort  VariantControl=Variant  PortDimensions=1
  EKF_depth : Subsystem
  EKF_position : Subsystem  TreatAsAtomicUnit=on
  hat_pos : Outport
  hat_depth : Outport  Port=2  PortDimensions=1
  flag_depth : Outport  Port=3  PortDimensions=1
  wires:
  orientation/1 -> EKF_position/3(orientation), EKF_depth/2(orientation)
  dvl/1 -> EKF_position/4(dvl), EKF_depth/3(dvl)
  depth_meas/1 -> EKF_depth/1(depth_meas)
  EKF_position/1(hat_pos) -> hat_pos/1
  EKF_depth/1(hat_depth) -> hat_depth/1
  EKF_depth/2(flag_depth) -> flag_depth/1
  orientation_flag/1 -> EKF_position/5(ahrs_flag), EKF_depth/4(ahrs_flag)
  GPS_flag/1 -> EKF_position/2(GPS_flag)
  meas_pos/1 -> EKF_position/1(meas_pos)
  dT/1 -> EKF_position/6(dT), EKF_depth/5(dT)
  init_pos/1 -> EKF_position/7(init_pos)
  P0_pos/1 -> EKF_position/8(P0_pos)
  init_depth/1 -> EKF_depth/6(init_depth)
  P0_depth/1 -> EKF_depth/7(P0_depth)

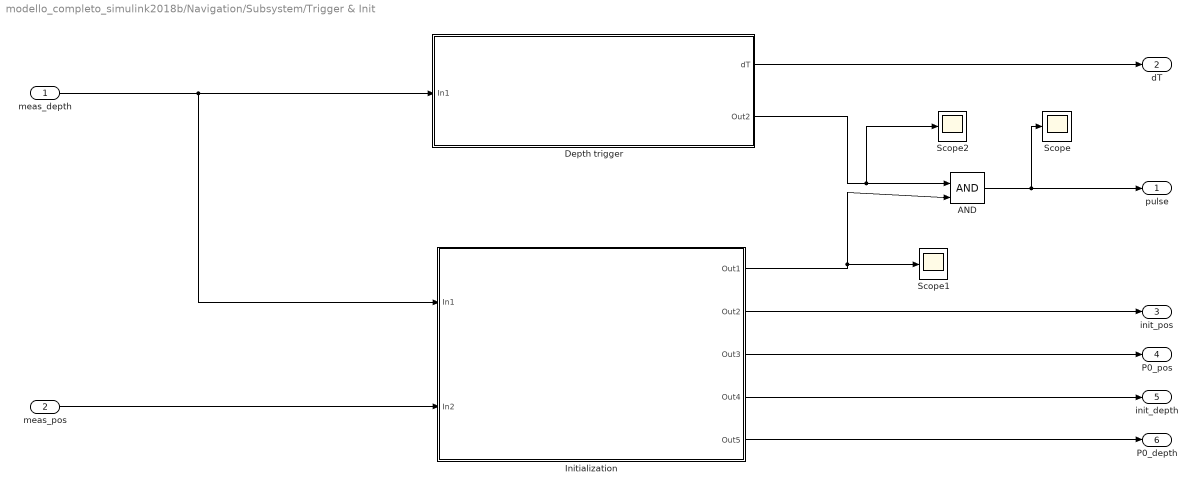
== system modello_completo_simulink2018b/Navigation/Subsystem/Trigger & Init ==
  meas_depth : Inport
  "meas_pos " : Inport  Port=2
  AND : Logic  IconShape=distinctive  AllPortsSameDT=off  OutDataTypeStr=boolean
  Depth trigger : Subsystem
  Initialization : Subsystem
  Scope : Scope
  Scope1 : Scope
  Scope2 : Scope
  pulse : Outport
  dT : Outport  Port=2
  init_pos : Outport  Port=3
  P0_pos : Outport  Port=4
  init_depth : Outport  Port=5
  P0_depth : Outport  Port=6
  wires:
  meas_depth/1 -> Depth trigger/1(In1), Initialization/1(In1)
  AND/1 -> Scope/1, pulse/1
  "meas_pos "/1 -> Initialization/2(In2)
  Initialization/2(Out2) -> init_pos/1
  Initialization/3(Out3) -> P0_pos/1
  Initialization/4(Out4) -> init_depth/1
  Initialization/5(Out5) -> P0_depth/1
  Depth trigger/1(dT) -> dT/1
  Depth trigger/2(Out2) -> Scope2/1, AND/1
  Initialization/1(Out1) -> Scope1/1, AND/2

== system modello_completo_simulink2018b/Vehicle Model/Model Vehicle/Kinematic ==
  eta : Inport
  ni : Inport  Port=2
  Jac : MATLAB Function  TreatAsAtomicUnit=on
  Product : Product  Multiplication=Matrix(*)
  eta_dot : Outport  VectorParamsAs1DForOutWhenUnconnected=off
  wires:
  ni/1 -> Product/2
  Jac/1(J) -> Product/1
  eta/1 -> Jac/1(eta)
  Product/1 -> eta_dot/1

== system modello_completo_simulink2018b/Vehicle Model/Thrusters/T ==
  des rot : Inport
  ni : Inport  Port=2
  Demux : Demux  Outputs=7
  Demux1 : Demux  Outputs=7
  MATLAB Function : MATLAB Function  TreatAsAtomicUnit=on
  Mux : Mux  Inputs=7
  Thruster 1 : Subsystem
  Thruster 2 : Subsystem
  Thruster 3 : Subsystem
  Thruster 4 : Subsystem
  Thruster 5 : Subsystem
  Thruster 6 : Subsystem
  Thruster 7 : Subsystem
  T : Outport  VectorParamsAs1DForOutWhenUnconnected=off
  wires:
  Demux/1 -> Thruster 1/1(n [rad/s])
  Demux/2 -> Thruster 2/1(n [rad/s])
  Demux/3 -> Thruster 3/1(n [rad/s])
  Demux/4 -> Thruster 4/1(n [rad/s])
  Demux/5 -> Thruster 5/1(n [rad/s])
  Demux/6 -> Thruster 6/1(n [rad/s])
  Demux/7 -> Thruster 7/1(n [rad/s])
  des rot/1 -> Demux/1
  Thruster 7/1(T i) -> Mux/7
  Thruster 6/1(T i) -> Mux/6
  Thruster 5/1(T i) -> Mux/5
  Thruster 4/1(T i) -> Mux/4
  Thruster 3/1(T i) -> Mux/3
  Thruster 2/1(T i) -> Mux/2
  Thruster 1/1(T i) -> Mux/1
  Mux/1 -> T/1
  MATLAB Function/1(v_th) -> Demux1/1
  Demux1/1 -> Thruster 1/2(V [m/s])
  Demux1/2 -> Thruster 2/2(V [m/s])
  Demux1/3 -> Thruster 3/2(V [m/s])
  Demux1/4 -> Thruster 4/2(V [m/s])
  Demux1/5 -> Thruster 5/2(V [m/s])
  Demux1/6 -> Thruster 6/2(V [m/s])
  Demux1/7 -> Thruster 7/2(V [m/s])
  ni/1 -> MATLAB Function/1(ni)

== system modello_completo_simulink2018b/Navigation/Subsystem/EKF/EKF_depth ==
  depth_meas : Inport
  orientation : Inport  Port=2
  dvl : Inport  Port=3
  ahrs_flag : Inport  Port=4
  dT : Inport  Port=5
  init_depth : Inport  Port=6
  P0_depth : Inport  Port=7
  Correzione : MATLAB Function  TreatAsAtomicUnit=on
  P_depth : Memory  InheritSampleTime=on  StateName=P_depth
  Predizione : MATLAB Function  TreatAsAtomicUnit=on
  hat__depth : Memory  InheritSampleTime=on  StateName=hat_depth
  hat_depth : Outport  PortDimensions=1
  flag_depth : Outport  Port=2  PortDimensions=1
  wires:
  Correzione/1(P_depth) -> P_depth/1
  Correzione/2(hat_depth) -> hat__depth/1, hat_depth/1
  Correzione/3(flag_depth) -> flag_depth/1
  hat__depth/1 -> Predizione/2("hat_depth ")
  P_depth/1 -> Predizione/1("P_depth ")
  orientation/1 -> Predizione/4(orientation)
  dvl/1 -> Predizione/5(dvl)
  depth_meas/1 -> Correzione/3(depth_meas)
  Predizione/2(hat_depth) -> Correzione/2("hat_depth ")
  Predizione/1(P_depth) -> Correzione/1("P_depth ")
  ahrs_flag/1 -> Predizione/8(ahrs_flag)
  dT/1 -> Predizione/3(dT)
  init_depth/1 -> Predizione/6(init_depth)
  P0_depth/1 -> Predizione/7(P0_depth)

== system modello_completo_simulink2018b/Navigation/Subsystem/EKF/EKF_position ==
  meas_pos : Inport
  GPS_flag : Inport  Port=2
  orientation : Inport  Port=3
  dvl : Inport  Port=4
  ahrs_flag : Inport  Port=5
  dT : Inport  Port=6
  init_pos : Inport  Port=7
  P0_pos : Inport  Port=8
  "Correzione " : MATLAB Function  TreatAsAtomicUnit=on
  P_pos : Memory  InitialCondition=zeros(2)  InheritSampleTime=on  StateName=P_pos
  Predizione : MATLAB Function  TreatAsAtomicUnit=on
  hat__pos : Memory  InitialCondition=zeros(2,1)  InheritSampleTime=on  StateName=P_pos
  previous_pos : Memory  InitialCondition=zeros(2,1)  InheritSampleTime=on  StateName=P_pos
  hat_pos : Outport
  wires:
  orientation/1 -> Predizione/4(orientation)
  hat__pos/1 -> Predizione/2("hat_pos ")
  previous_pos/1 -> "Correzione "/1("prev_pos ")
  Predizione/2(hat_pos) -> "Correzione "/3("hat_pos ")
  "Correzione "/1(prev_pos) -> previous_pos/1
  dvl/1 -> Predizione/5(dvl)
  P_pos/1 -> Predizione/1("P_pos ")
  GPS_flag/1 -> "Correzione "/5(GPS_flag)
  ahrs_flag/1 -> Predizione/6(ahrs_flag)
  "Correzione "/2(P_pos) -> P_pos/1
  "Correzione "/3(hat_pos) -> hat__pos/1, hat_pos/1
  meas_pos/1 -> "Correzione "/4(meas_pos)
  Predizione/1(P_pos) -> "Correzione "/2("P_pos ")
  dT/1 -> Predizione/3(dT)
  init_pos/1 -> Predizione/7(init_pos)
  P0_pos/1 -> Predizione/8(P0_pos)

== system modello_completo_simulink2018b/Navigation/Subsystem/Trigger & Init/Depth trigger ==
  In1 : Inport
  Demux : Demux  Outputs=2
  MATLAB Function : MATLAB Function  TreatAsAtomicUnit=on  SystemSampleTime=1/200
  Scope2 : Scope
  Sum : Sum  Inputs=|+-
  Terminator : Terminator
  count : Memory
  prev_depth : Memory
  dT : Outport
  Out2 : Outport  Port=2
  wires:
  Sum/1 -> MATLAB Function/3(sum)
  prev_depth/1 -> Sum/2
  MATLAB Function/3(pulse) -> Scope2/1, Out2/1
  Demux/2 -> Terminator/1
  MATLAB Function/4(prev) -> prev_depth/1
  MATLAB Function/2(dT) -> dT/1
  In1/1 -> Demux/1
  count/1 -> MATLAB Function/1("count ")
  Demux/1 -> MATLAB Function/2(depth), Sum/1
  MATLAB Function/1(count) -> count/1

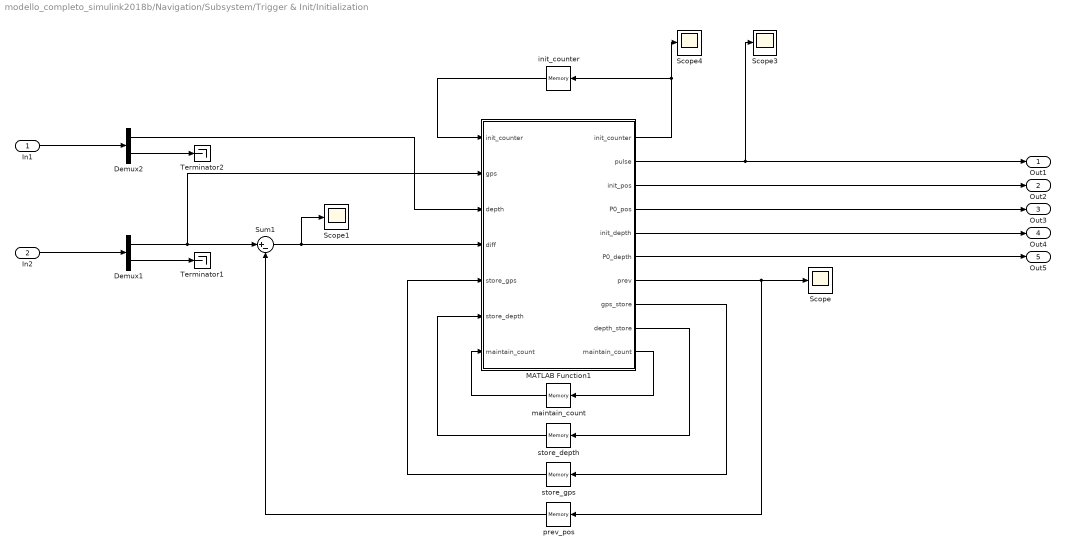
== system modello_completo_simulink2018b/Navigation/Subsystem/Trigger & Init/Initialization ==
  In1 : Inport
  In2 : Inport  Port=2
  Demux1 : Demux  Outputs=[2 1]
  Demux2 : Demux  Outputs=2
  MATLAB Function1 : MATLAB Function  TreatAsAtomicUnit=on  SystemSampleTime=1/200
  Scope{,1,3..4} (4 alike) : Scope
  Sum1 : Sum  Inputs=|+-
  Terminator1 : Terminator
  Terminator2 : Terminator
  init_counter : Memory
  maintain_count : Memory
  prev_pos : Memory  InitialCondition=zeros(2,1)
  store_depth : Memory  InitialCondition=zeros(5,1)
  store_gps : Memory  InitialCondition=zeros(2,5)
  Out1 : Outport
  Out2 : Outport  Port=2
  Out3 : Outport  Port=3
  Out4 : Outport  Port=4
  Out5 : Outport  Port=5
  wires:
  Demux1/1 -> MATLAB Function1/2(gps), Sum1/1
  MATLAB Function1/4(P0_pos) -> Out3/1
  MATLAB Function1/3(init_pos) -> Out2/1
  MATLAB Function1/2(pulse) -> Scope3/1, Out1/1
  init_counter/1 -> MATLAB Function1/1("init_counter ")
  Sum1/1 -> Scope1/1, MATLAB Function1/4(diff)
  MATLAB Function1/10(maintain_count) -> maintain_count/1
  Demux2/1 -> MATLAB Function1/3(depth)
  MATLAB Function1/8(gps_store) -> store_gps/1
  maintain_count/1 -> MATLAB Function1/7("maintain_count ")
  MATLAB Function1/1(init_counter) -> Scope4/1, init_counter/1
  Demux2/2 -> Terminator2/1
  MATLAB Function1/9(depth_store) -> store_depth/1
  store_gps/1 -> MATLAB Function1/5(store_gps)
  store_depth/1 -> MATLAB Function1/6(store_depth)
  In1/1 -> Demux2/1
  MATLAB Function1/7(prev) -> prev_pos/1, Scope/1
  prev_pos/1 -> Sum1/2
  Demux1/2 -> Terminator1/1
  In2/1 -> Demux1/1
  MATLAB Function1/6(P0_depth) -> Out5/1
  MATLAB Function1/5(init_depth) -> Out4/1

== system modello_completo_simulink2018b/Vehicle Model/Thrusters/T/Thruster 1 ==
  note: n is the rotational speed of the thruster
      | V is the speed component of the water along the thruster axis
      |
      | n is saturated according to data
      | a dead zone is considered according to data
      | the thruster is characterised by 1st order dynamics (tau = 0.2s)
  n [rad/s] : Inport
  V [m/s] : Inport  Port=2
  Dead Zone : DeadZone  LowerValue=-dead_zone_limit  UpperValue=dead_zone_limit  SaturateOnIntegerOverflow=on
  MATLAB Function : MATLAB Function  TreatAsAtomicUnit=on
  Saturation : Saturate  UpperLimit=n_max  LowerLimit=-n_max
  Transfer Fcn : TransferFcn  Denominator=[0.2 1]
  T i : Outport
  wires:
  V [m/s]/1 -> MATLAB Function/2(V)
  Saturation/1 -> MATLAB Function/1(n)
  Transfer Fcn/1 -> Saturation/1
  Dead Zone/1 -> Transfer Fcn/1
  n [rad/s]/1 -> Dead Zone/1
  MATLAB Function/1(T) -> T i/1

== system modello_completo_simulink2018b/Vehicle Model/Thrusters/T/Thruster 2 ==
  note: n is the rotational speed of the thruster
      | V is the speed component of the water along the thruster axis
      |
      | n is saturated according to data
      | a dead zone is considered according to data
      | the thruster is characterised by 1st order dynamics (tau = 0.2s)
  n [rad/s] : Inport
  V [m/s] : Inport  Port=2
  Dead Zone : DeadZone  LowerValue=-dead_zone_limit  UpperValue=dead_zone_limit  SaturateOnIntegerOverflow=on
  MATLAB Function : MATLAB Function  TreatAsAtomicUnit=on
  Saturation : Saturate  UpperLimit=n_max  LowerLimit=-n_max
  Transfer Fcn : TransferFcn  Denominator=[0.2 1]
  T i : Outport
  wires:
  V [m/s]/1 -> MATLAB Function/2(V)
  Saturation/1 -> MATLAB Function/1(n)
  Transfer Fcn/1 -> Saturation/1
  Dead Zone/1 -> Transfer Fcn/1
  n [rad/s]/1 -> Dead Zone/1
  MATLAB Function/1(T) -> T i/1

== system modello_completo_simulink2018b/Vehicle Model/Thrusters/T/Thruster 3 ==
  note: n is the rotational speed of the thruster
      | V is the speed component of the water along the thruster axis
      |
      | n is saturated according to data
      | a dead zone is considered according to data
      | the thruster is characterised by 1st order dynamics (tau = 0.2s)
  n [rad/s] : Inport
  V [m/s] : Inport  Port=2
  Dead Zone : DeadZone  LowerValue=-dead_zone_limit  UpperValue=dead_zone_limit  SaturateOnIntegerOverflow=on
  MATLAB Function : MATLAB Function  TreatAsAtomicUnit=on
  Saturation : Saturate  UpperLimit=n_max  LowerLimit=-n_max
  Transfer Fcn : TransferFcn  Denominator=[0.2 1]
  T i : Outport
  wires:
  V [m/s]/1 -> MATLAB Function/2(V)
  Saturation/1 -> MATLAB Function/1(n)
  Transfer Fcn/1 -> Saturation/1
  Dead Zone/1 -> Transfer Fcn/1
  n [rad/s]/1 -> Dead Zone/1
  MATLAB Function/1(T) -> T i/1

== system modello_completo_simulink2018b/Vehicle Model/Thrusters/T/Thruster 4 ==
  note: n is the rotational speed of the thruster
      | V is the speed component of the water along the thruster axis
      |
      | n is saturated according to data
      | a dead zone is considered according to data
      | the thruster is characterised by 1st order dynamics (tau = 0.2s)
  n [rad/s] : Inport
  V [m/s] : Inport  Port=2
  Dead Zone : DeadZone  LowerValue=-dead_zone_limit  UpperValue=dead_zone_limit  SaturateOnIntegerOverflow=on
  MATLAB Function : MATLAB Function  TreatAsAtomicUnit=on
  Saturation : Saturate  UpperLimit=n_max  LowerLimit=-n_max
  Transfer Fcn : TransferFcn  Denominator=[0.2 1]
  T i : Outport
  wires:
  V [m/s]/1 -> MATLAB Function/2(V)
  Saturation/1 -> MATLAB Function/1(n)
  Transfer Fcn/1 -> Saturation/1
  Dead Zone/1 -> Transfer Fcn/1
  n [rad/s]/1 -> Dead Zone/1
  MATLAB Function/1(T) -> T i/1

== system modello_completo_simulink2018b/Vehicle Model/Thrusters/T/Thruster 5 ==
  note: n is the rotational speed of the thruster
      | V is the speed component of the water along the thruster axis
      |
      | n is saturated according to data
      | a dead zone is considered according to data
      | the thruster is characterised by 1st order dynamics (tau = 0.2s)
  n [rad/s] : Inport
  V [m/s] : Inport  Port=2
  Dead Zone : DeadZone  LowerValue=-dead_zone_limit  UpperValue=dead_zone_limit  SaturateOnIntegerOverflow=on
  MATLAB Function : MATLAB Function  TreatAsAtomicUnit=on
  Saturation : Saturate  UpperLimit=n_max  LowerLimit=-n_max
  Transfer Fcn : TransferFcn  Denominator=[0.2 1]
  T i : Outport
  wires:
  V [m/s]/1 -> MATLAB Function/2(V)
  Saturation/1 -> MATLAB Function/1(n)
  Transfer Fcn/1 -> Saturation/1
  Dead Zone/1 -> Transfer Fcn/1
  n [rad/s]/1 -> Dead Zone/1
  MATLAB Function/1(T) -> T i/1

== system modello_completo_simulink2018b/Vehicle Model/Thrusters/T/Thruster 6 ==
  note: n is the rotational speed of the thruster
      | V is the speed component of the water along the thruster axis
      |
      | n is saturated according to data
      | a dead zone is considered according to data
      | the thruster is characterised by 1st order dynamics (tau = 0.2s)
  n [rad/s] : Inport
  V [m/s] : Inport  Port=2
  Dead Zone : DeadZone  LowerValue=-dead_zone_limit  UpperValue=dead_zone_limit  SaturateOnIntegerOverflow=on
  MATLAB Function : MATLAB Function  TreatAsAtomicUnit=on
  Saturation : Saturate  UpperLimit=n_max  LowerLimit=-n_max
  Transfer Fcn : TransferFcn  Denominator=[0.2 1]
  T i : Outport
  wires:
  V [m/s]/1 -> MATLAB Function/2(V)
  Saturation/1 -> MATLAB Function/1(n)
  Transfer Fcn/1 -> Saturation/1
  Dead Zone/1 -> Transfer Fcn/1
  n [rad/s]/1 -> Dead Zone/1
  MATLAB Function/1(T) -> T i/1

== system modello_completo_simulink2018b/Vehicle Model/Thrusters/T/Thruster 7 ==
  note: n is the rotational speed of the thruster
      | V is the speed component of the water along the thruster axis
      |
      | n is saturated according to data
      | a dead zone is considered according to data
      | the thruster is characterised by 1st order dynamics (tau = 0.2s)
  n [rad/s] : Inport
  V [m/s] : Inport  Port=2
  Dead Zone : DeadZone  LowerValue=-dead_zone_limit  UpperValue=dead_zone_limit  SaturateOnIntegerOverflow=on
  MATLAB Function : MATLAB Function  TreatAsAtomicUnit=on
  Saturation : Saturate  UpperLimit=n_max  LowerLimit=-n_max
  Transfer Fcn : TransferFcn  Denominator=[0.2 1]
  T i : Outport
  wires:
  V [m/s]/1 -> MATLAB Function/2(V)
  Saturation/1 -> MATLAB Function/1(n)
  Transfer Fcn/1 -> Saturation/1
  Dead Zone/1 -> Transfer Fcn/1
  n [rad/s]/1 -> Dead Zone/1
  MATLAB Function/1(T) -> T i/1

== matlab function modello_completo_simulink2018b/Vehicle Model/Model Vehicle/D ==
  data: ni_r input; F_d output; rho input
function F_d = D_forces(ni_r, rho)
    ni_lin = ni_r(1:3);
    ni_ang = ni_r(4:6);
    a = 0.35;
    b = a;
    c = 0.19;
    A_ab = pi*a*b;      % moto lin lungo z; rotatorio intorno a x e y
    A_bc = pi*b*c;      % moto lin lungo x; rotatorio intorno a z
    A_ac = pi*a*c;      % moto lin lungo y
%     C_d  =  0.0489;
%     D_coeff = -1/2*rho*C_d*diag([A_bc, A_ac, A_ab, A_bc, A_ac, A_ab]);
%     F_d = D_coeff*(abs(ni_r).*ni_r);
    visc = 0.001;       % Pa*s (per una temperatura di 20° e rho = 1030)
    vmax = 0.3;
    Di = 0.7;
    Re = Di/(visc/rho)*vmax; % Re = 2*1e5
    Cd = 0.49;
    rm_z = 4*c/(3*pi);
    rm_xy = 4*a/(3*pi);
    D_lin = -1/2*rho*Cd*diag([A_bc, A_ac, A_ab])*(abs(ni_lin).*ni_lin);
    D_ang = -1/2*rho*Cd*diag([rm_xy^3*A_ab, rm_xy^3*A_ab, rm_z^3*A_bc])*(abs(ni_ang).*ni_ang);
    F_d = [D_lin; D_ang];
end

== matlab function modello_completo_simulink2018b/Vehicle Model/Model Vehicle/C ==
  data: ni_r input; F_c output; M input
function F_c = C(ni_r, M)
    ni = ni_r;
    M11 = M(1:3,1:3);
    M22 = M(4:6,4:6);
    ni1 = ni(1:3);
    ni2 = ni(4:6);
    C11 = zeros(3,3);
    s1 = M11*ni1;
    C12 = - [0 -s1(3) s1(2); s1(3) 0 -s1(1); -s1(2) s1(1) 0];
    C21 = C12;
    s2 = M22*ni2;
    C22 = - [0 -s2(3) s2(2); s2(3) 0 -s2(1); -s2(2) s2(1) 0];
    F_c = [C11 C12; C21 C22]*ni_r;
end
